simulink model "WESDem_StrtBtnSP"  (R2016b)
settings: configuration reference "CodeGenConfigSet" (kept outside this file)
values from neighbouring files (symbols this model uses):
  WESDem_dnStrtBtnSPRmpDwn_C = Calibration.Parameter    [init_WESDem_StrtBtnSP.m]
  WESDem_dnStrtBtnSPRmpUp_C = Calibration.Parameter    [init_WESDem_StrtBtnSP.m]
  WESDem_nStrtBtnLim_C = Calibration.Parameter    [init_WESDem_StrtBtnSP.m]
  WESDem_stActvCond_C = Calibration.Parameter    [init_WESDem_StrtBtnSP.m]
  WESDem_vStrtBtnActv_C = Calibration.Parameter    [init_WESDem_StrtBtnSP.m]
undefined symbols (not defined in the file or in its folder): StSys_StrtState_conv, Switch_conv, WESDem_State_conv
libraries: CXLib x9
settings Model: Creator=zhoukai  LastModifiedBy=zhoukai
settings ConfigSetRef: SourceLocation=Base Workspace

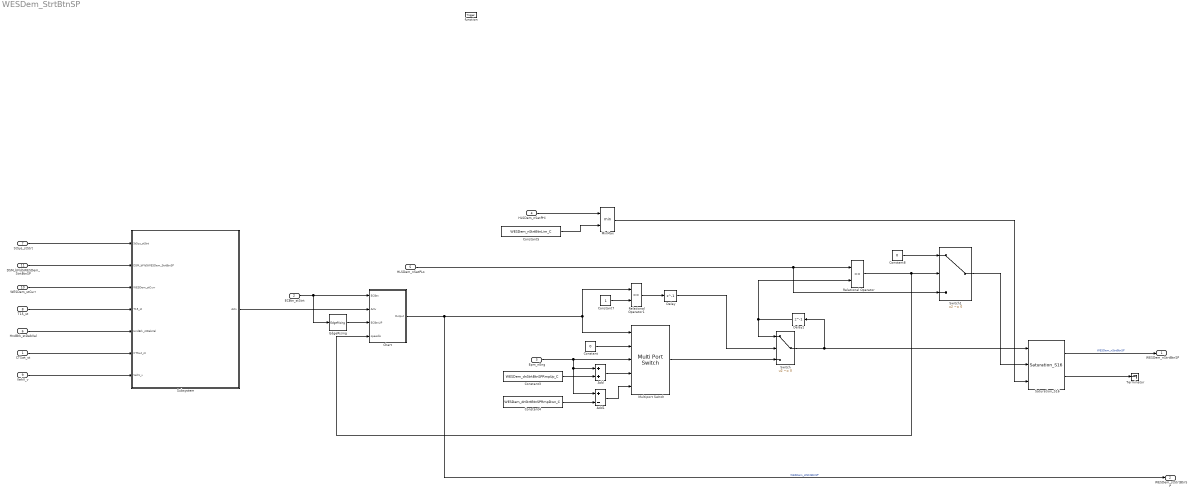
== system WESDem_StrtBtnSP ==
  CTSwt_st : Inport  Description=Status of cabin tilt switch component driver  OutMin=0  OutMax=1  OutDataTypeStr=boolean
  ECBtn_stStrt : Inport  Description=Start Button state for ECBtn  Port=2  OutMin=0  OutMax=1  OutDataTypeStr=boolean
  Epm_nEng : Inport  Tag=rpm  Description=Engine speed  Port=3  OutMin=0  OutMax=6000  OutDataTypeStr=EngSpeed_rpm
  HLSDem_nSetPHi : Inport  Tag=rpm  Description=Maximum engine speed of HLSDem  Port=4  OutMin=0  OutMax=6000  OutDataTypeStr=EngSpeed_rpm
  HLSDem_nSetPLo : Inport  Tag=rpm  Description=Minimum engine speed of HLSDem  Port=5  OutMin=0  OutMax=6000  OutDataTypeStr=EngSpeed_rpm
  HndBrk_stDebVal : Inport  Description=Debounced value of Hand Brake switch  Port=6  OutMin=0  OutMax=255  OutDataTypeStr=State_uint8
  StSys_stStrt : Inport  Description=State of starting system  Port=7  OutDataTypeStr=Enum: StSys_StrtState_conv
  T15_st : Inport  Description=Terminal 15 status after denouncing  Port=8  OutDataTypeStr=Enum: Switch_conv
  VehV_v : Inport  Tag=km/h  Description=Vehicle speed  Port=9  OutMin=0  OutMax=250  OutDataTypeStr=VehSpeed_km_h
  WESDem_stCurr : Inport  Description=Status of the working engine Speed Control  Port=10  OutDataTypeStr=Enum: WESDem_State_conv
  DSM_bFld5WESDem_StrtBtnSP : Inport  Description=FId inhibits if WESDem start button is faulty  Port=11  OutMin=0  OutMax=1  OutDataTypeStr=boolean
  function : TriggerPort  TriggerType=function-call  VariantControl=Variant
  Add : Sum
  Add1 : Sum  Inputs=+-
  Chart : Stateflow chart  TreatAsAtomicUnit=on
  Constant : Constant  Value=0  OutDataTypeStr=Inherit: Inherit via back propagation
  Constant3 : Constant  Value=WESDem_dnStrtBtnSPRmpUp_C
  Constant4 : Constant  Value=WESDem_dnStrtBtnSPRmpDwn_C
  Constant5 : Constant  Value=WESDem_nStrtBtnLim_C
  Constant7 : Constant  OutDataTypeStr=Inherit: Inherit via back propagation
  Constant8 : Constant  Value=0  OutDataTypeStr=Inherit: Inherit via back propagation
  Delay : Delay  DelayLength=1
  Delay1 : Delay  DelayLength=1
  EdgeRising : CXLib/EdgeRising
  MinMax : MinMax  Inputs=2
  Multiport Switch : MultiPortSwitch  DataPortOrder=Zero-based contiguous  Inputs=4
  Relational Operator : RelationalOperator  OutDataTypeStr=boolean  RndMeth=Simplest
  Relational Operator1 : RelationalOperator  Operator===  OutDataTypeStr=boolean  RndMeth=Simplest
  Saturation_S16 : CXLib/Saturation_S16
  Subsystem : Subsystem
  Switch : Switch  Criteria=u2 ~= 0
  Switch1 : Switch  Criteria=u2 ~= 0
  Terminator : Terminator
  WESDem_nStrtBtnSP : Outport  Tag=rpm  Description=Working engine speed setpoint through start button  OutMin=0  OutMax=6000  OutDataTypeStr=EngSpeed_rpm
  WESDem_stStrtBtnSP : Outport  Description=Status of working engine speed setpoint through start button  Port=2  OutMin=0  OutMax=255  OutDataTypeStr=State_uint8
  wires:
  Epm_nEng/1 -> Add1/1, Add/1, Multiport Switch/3
  Constant/1 -> Multiport Switch/2
  Add/1 -> Multiport Switch/4
  Constant3/1 -> Add/2
  Constant4/1 -> Add1/2
  Add1/1 -> Multiport Switch/5
  HLSDem_nSetPHi/1 -> MinMax/1
  Constant5/1 -> MinMax/2
  HLSDem_nSetPLo/1 -> Switch1/3, Relational Operator/1
  Chart/1(Output) -> WESDem_stStrtBtnSP/1, Multiport Switch/1, Relational Operator1/1  "WESDem_stStrtBtnSP"
  Relational Operator1/1 -> Delay/1
  Constant7/1 -> Relational Operator1/2
  Delay/1 -> Switch/2
  Constant8/1 -> Switch1/1
  Switch1/1 -> Saturation_S16/2
  MinMax/1 -> Saturation_S16/3
  Subsystem/1(Actv) -> Chart/2(Actv)
  ECBtn_stStrt/1 -> EdgeRising/1, Chart/1(ECBtn)
  EdgeRising/1 -> Chart/3(ECBtnUP)
  Saturation_S16/1 -> WESDem_nStrtBtnSP/1  "WESDem_nStrtBtnSP"
  Saturation_S16/2 -> Terminator/1
  VehV_v/1 -> Subsystem/7("VehV_v ")
  T15_st/1 -> Subsystem/4(T15_st)
  CTSwt_st/1 -> Subsystem/6(CTSwt_st)
  HndBrk_stDebVal/1 -> Subsystem/5(HndBrk_stDebVal)
  WESDem_stCurr/1 -> Subsystem/3(WESDem_stCurr)
  StSys_stStrt/1 -> Subsystem/1(StSys_stStrt)
  DSM_bFld5WESDem_StrtBtnSP/1 -> Subsystem/2(DSM_bFld5WESDem_StrtBtnSP)
  Relational Operator/1 -> Chart/4(speedlo), Switch1/2
  Switch/1 -> Delay1/1, Saturation_S16/1
  Multiport Switch/1 -> Switch/3
  Delay1/1 -> Switch/1, Relational Operator/2

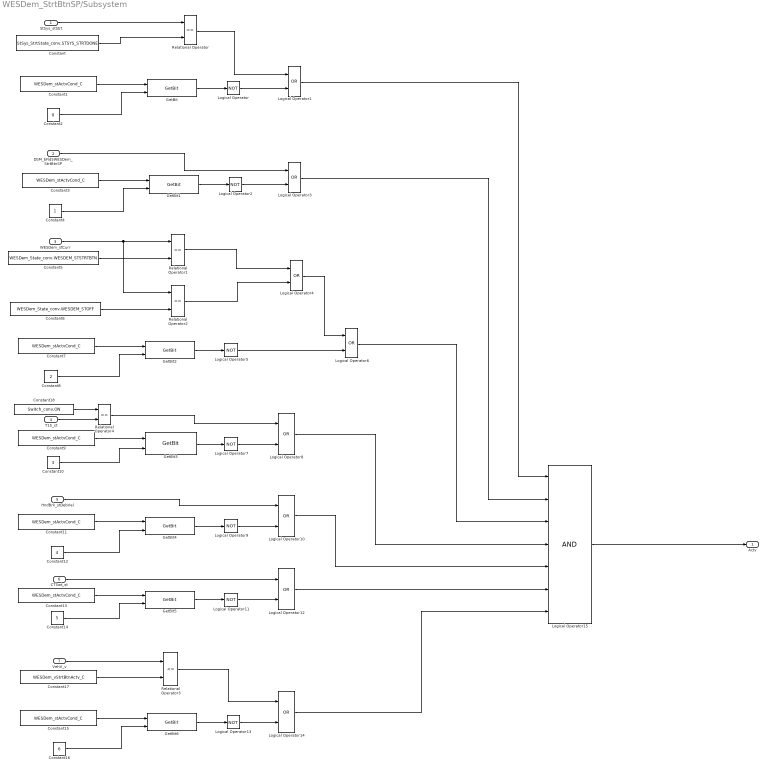
== system WESDem_StrtBtnSP/Subsystem ==
  StSys_stStrt : Inport
  DSM_bFld5WESDem_StrtBtnSP : Inport  Port=2
  WESDem_stCurr : Inport  Port=3
  T15_st : Inport  Port=4
  HndBrk_stDebVal : Inport  Port=5
  CTSwt_st : Inport  Port=6
  "VehV_v " : Inport  Port=7
  Constant : Constant  Value=StSys_StrtState_conv.STSYS_STRTDONE  OutDataTypeStr=Inherit: Inherit via back propagation
  Constant{1,3,7,9,11,13,15} (7 alike) : Constant  Value=WESDem_stActvCond_C
  Constant10 : Constant  Value=3  OutDataTypeStr=Inherit: Inherit via back propagation
  Constant12 : Constant  Value=4  OutDataTypeStr=Inherit: Inherit via back propagation
  Constant14 : Constant  Value=5  OutDataTypeStr=Inherit: Inherit via back propagation
  Constant16 : Constant  Value=6  OutDataTypeStr=Inherit: Inherit via back propagation
  Constant17 : Constant  Value=WESDem_vStrtBtnActv_C
  Constant18 : Constant  Value=Switch_conv.ON
  Constant2 : Constant  Value=0  OutDataTypeStr=Inherit: Inherit via back propagation
  Constant4 : Constant  OutDataTypeStr=Inherit: Inherit via back propagation
  Constant5 : Constant  Value=WESDem_State_conv.WESDEM_STSTRTBTN
  Constant6 : Constant  Value=WESDem_State_conv.WESDEM_STOFF
  Constant8 : Constant  Value=2  OutDataTypeStr=Inherit: Inherit via back propagation
  GetBit{,1..6} (7 alike) : CXLib/GetBit  dataTypeString=uint8  dataLength=0
      settings: AttributesFormatString=Get bit from %<dataTypeString>
  Logical Operator{,2,5,7,9,11,13} (7 alike) : Logic  Operator=NOT  AllPortsSameDT=off  OutDataTypeStr=boolean
  Logical Operator{1,3..4,6,8,10,12,14} (8 alike) : Logic  Operator=OR  AllPortsSameDT=off  OutDataTypeStr=boolean
  Logical Operator15 : Logic  Inputs=7  AllPortsSameDT=off  OutDataTypeStr=boolean
  Relational Operator{,1..2,4} (4 alike) : RelationalOperator  Operator===  OutDataTypeStr=boolean  RndMeth=Simplest
  Relational Operator3 : RelationalOperator  Operator=<=  OutDataTypeStr=boolean  RndMeth=Simplest
  Actv : Outport
  wires:
  StSys_stStrt/1 -> Relational Operator/1
  Constant/1 -> Relational Operator/2
  Constant1/1 -> GetBit/1
  Constant2/1 -> GetBit/2
  GetBit/1 -> Logical Operator/1
  Relational Operator/1 -> Logical Operator1/1
  Logical Operator/1 -> Logical Operator1/2
  Constant3/1 -> GetBit1/1
  Constant4/1 -> GetBit1/2
  GetBit1/1 -> Logical Operator2/1
  Logical Operator2/1 -> Logical Operator3/2
  DSM_bFld5WESDem_StrtBtnSP/1 -> Logical Operator3/1
  Constant5/1 -> Relational Operator1/2
  WESDem_stCurr/1 -> Relational Operator2/1, Relational Operator1/1
  Constant6/1 -> Relational Operator2/2
  Relational Operator1/1 -> Logical Operator4/1
  Relational Operator2/1 -> Logical Operator4/2
  Constant7/1 -> GetBit2/1
  Constant8/1 -> GetBit2/2
  GetBit2/1 -> Logical Operator5/1
  Logical Operator5/1 -> Logical Operator6/2
  Logical Operator4/1 -> Logical Operator6/1
  Constant9/1 -> GetBit3/1
  Constant10/1 -> GetBit3/2
  GetBit3/1 -> Logical Operator7/1
  Logical Operator7/1 -> Logical Operator8/2
  Constant11/1 -> GetBit4/1
  Constant12/1 -> GetBit4/2
  GetBit4/1 -> Logical Operator9/1
  Logical Operator9/1 -> Logical Operator10/2
  HndBrk_stDebVal/1 -> Logical Operator10/1
  Constant13/1 -> GetBit5/1
  Constant14/1 -> GetBit5/2
  GetBit5/1 -> Logical Operator11/1
  Logical Operator11/1 -> Logical Operator12/2
  CTSwt_st/1 -> Logical Operator12/1
  Constant15/1 -> GetBit6/1
  Constant16/1 -> GetBit6/2
  GetBit6/1 -> Logical Operator13/1
  Logical Operator13/1 -> Logical Operator14/2
  Constant17/1 -> Relational Operator3/2
  "VehV_v "/1 -> Relational Operator3/1
  Relational Operator3/1 -> Logical Operator14/1
  Logical Operator1/1 -> Logical Operator15/1
  Logical Operator3/1 -> Logical Operator15/2
  Logical Operator6/1 -> Logical Operator15/3
  Logical Operator8/1 -> Logical Operator15/4
  Logical Operator10/1 -> Logical Operator15/5
  Logical Operator12/1 -> Logical Operator15/6
  Logical Operator14/1 -> Logical Operator15/7
  Logical Operator15/1 -> Actv/1
  T15_st/1 -> Relational Operator4/2
  Constant18/1 -> Relational Operator4/1
  Relational Operator4/1 -> Logical Operator8/1

== stateflow chart WESDem_StrtBtnSP/Chart ==
  state WESDEM_STSTRTBTNOFF
    entry:Output=uint8(0);
  state WESDEM_STSTRTBTNRMPDWN
    entry:Output=uint8(3);
  state WESDEM_STSTRTBTNRMPUP
    entry:Output=uint8(2);
  state WESDEM_STSTRTBTNNEUTRAL
    entry:Output=uint8(1);
  (default) -> WESDEM_STSTRTBTNOFF
  WESDEM_STSTRTBTNRMPDWN -> WESDEM_STSTRTBTNOFF [order 1] : [Actv==0]
  WESDEM_STSTRTBTNRMPUP -> WESDEM_STSTRTBTNOFF [order 1] : [Actv==0]
  WESDEM_STSTRTBTNOFF -> WESDEM_STSTRTBTNRMPUP [order 1] : [Actv==1&&speedlo==1&&ECBtn==1&&ECBtnUP==1]
  WESDEM_STSTRTBTNNEUTRAL -> WESDEM_STSTRTBTNOFF [order 1] : [Actv==0]
  WESDEM_STSTRTBTNOFF -> WESDEM_STSTRTBTNRMPDWN [order 2] : [Actv==1&&speedlo==0&&ECBtn==1&&ECBtnUP==1]
  WESDEM_STSTRTBTNRMPDWN -> WESDEM_STSTRTBTNNEUTRAL [order 2] : [ECBtn==0]
  WESDEM_STSTRTBTNNEUTRAL -> WESDEM_STSTRTBTNRMPDWN [order 3] : [ECBtn==1&&speedlo==1]
  WESDEM_STSTRTBTNNEUTRAL -> WESDEM_STSTRTBTNRMPUP [order 2] : [ECBtn==1&&speedlo==0]
  WESDEM_STSTRTBTNRMPUP -> WESDEM_STSTRTBTNNEUTRAL [order 2] : [ECBtn==0]
  data: Output output; ECBtn input; Actv input; ECBtnUP input; speedlo input
